simulink model "Copy_of_InvertedPendulumSimLuenberger"  (Simulink 9.2)
settings: Solver=ode5  StartTime=0.0  StopTime=30  FixedStep=0.01  RelTol=1e-3  AbsTol=1e-6
PreLoadFcn:
  | InvertedPendulumSimLuenbergerInit
InitFcn:
  | clear PlotPendulum
values from neighbouring files (symbols this model uses):
  A = [0, 1,          0,              0 ... (first row only)    [InvertedPendulumSimLuenbergerInit.m]    (also in aufgabe81.m = [0, -1; 1, -2]; aufgabe82.m = [0, 1; -1, 1])
  B = [ 0; J/d; 0; -mp*l/d]    [InvertedPendulumSimLuenbergerInit.m]    (also in aufgabe81.m = [0; 0.5]; aufgabe82.m = [0; 0.5])
  C = [ 1 0 0 0 ... (first row only)    [InvertedPendulumSimLuenbergerInit.m]    (also in aufgabe81.m = [0, 1]; aufgabe82.m = [1, 0])
  eta = 1.05    [InvertedPendulumSimLuenbergerInit.m]
  K = place(A,B,poles)    [InvertedPendulumSimLuenbergerInit.m]    (also in aufgabe82.m = place(A, B, [-3, -4]))
  kcw = 3    [InvertedPendulumSimLuenbergerInit.m]
  kem = 7    [InvertedPendulumSimLuenbergerInit.m]
  ksu = 1.3    [InvertedPendulumSimLuenbergerInit.m]
  kvw = 3    [InvertedPendulumSimLuenbergerInit.m]
  L = place(A', C', 2 * poles)'    [InvertedPendulumSimLuenbergerInit.m]    (also in aufgabe81.m = Lt'; aufgabe82.m = Lt')
  sigmaCart = 0    [InvertedPendulumSimLuenbergerInit.m]
  sigmaPend = 0    [InvertedPendulumSimLuenbergerInit.m]
  Td = 0    [InvertedPendulumSimLuenbergerInit.m]
  vmax = 5    [InvertedPendulumSimLuenbergerInit.m]
  x0 = [0; 0; pi-0.01; 0]    [InvertedPendulumSimLuenbergerInit.m]    (also in aufgabe81.m = [ -1; 1]; aufgabe82.m = [ -1; 1])
  x0hat = [0; 0; pi; 0]    [InvertedPendulumSimLuenbergerInit.m]    (also in aufgabe81.m = [ -2; 2]; aufgabe82.m = [ -2; 2])
  xmax = 0.4    [InvertedPendulumSimLuenbergerInit.m]
undefined symbols (not defined in the file or in its folder): fc, fp, Fs, g, J, l, M, m, mp, PlotPendulum, sgn, Ts
undefined symbols (not defined in the file): angleSZ
libraries: simulink x2
settings Model: LogicAnalyzerSignalOrdering=3f8627a9-a3d2-4771-9af9-cb62c719a4c2,aa08fdaf-5472-4d0b-8e2c-dcdd649b45f6,f94730cb-f55a-4896-8059-4683a2930ab6,1e4896a6-91b5-40dd-8c6c-ecf390694b00  Creator=jims  LastModifiedBy=root  ExtModeTrigDuration=12000  ExtModeTrigLevel=0.400000
settings SolverCC: AutoScaleAbsTol=off
settings DataIOCC: ExternalInput=[]  InitialState=[]  LimitDataPoints=off  MaxDataPoints=5000  SignalLoggingSaveFormat=Dataset  SaveOutput=off  SaveTime=off  SignalLoggingName=sigsOut
settings OptimizationCC: BooleanDataType=off  InitFltsAndDblsToZero=on
settings DebuggingCC: SaveWithParameterizedLinksMsg=none  SignalResolutionControl=TryResolveAllWithWarning  MultiTaskDSMMsg=warning  MultiTaskCondExecSysMsg=none  IntegerOverflowMsg=none  StateNameClashWarn=none  IntegerSaturationMsg=none
settings HardwareCC: TargetBitPerLong=64  TargetBitPerPointer=64  TargetBitPerSizeT=64  TargetBitPerPtrDiffT=64  TargetLongLongMode=on  TargetIntDivRoundTo=Zero  TargetEndianess=LittleEndian  TargetWordSize=64  TargetHWDeviceType=MATLAB Host  ProdEqTarget=off
settings SFSimCC: SimUseLocalCustomCode=on  SimParseCustomCode=off
settings RTWCC: SystemTargetFile=rtwin.tlc  TemplateMakefile=rtwin.tmf  RTWUseLocalCustomCode=on
settings TargetCC: TargetFcnLib=ansi_tfl_tmw.mat  ModelReferenceCompliant=off  CompOptLevelCompliant=off  GeneratePreprocessorConditionals=Use local settings  PreserveStateflowLocalDataDimensions=off
settings CustomProperty: DataType=string  Value=on
settings ConfigComp: CovExternalEMLEnable=on

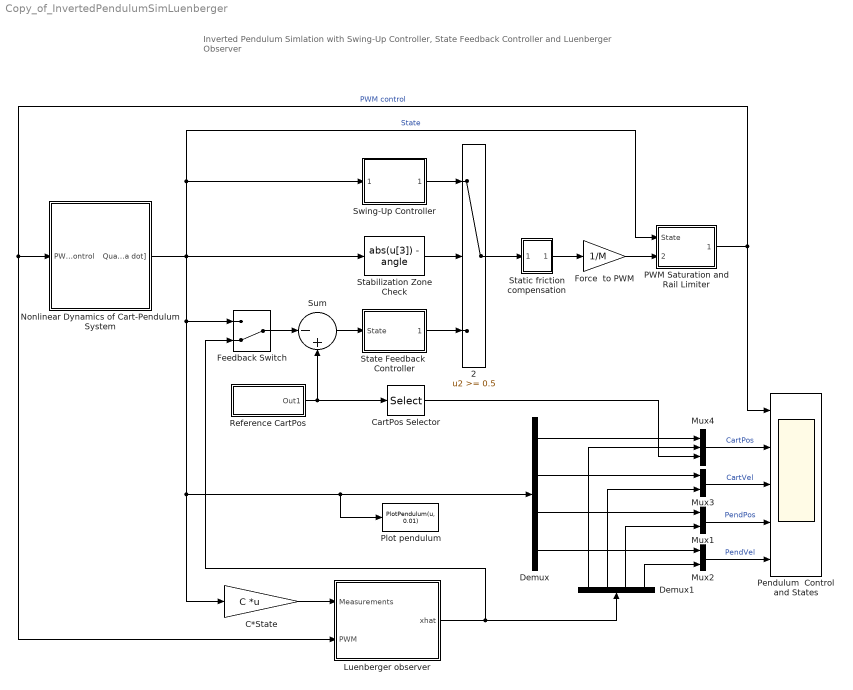
== system Copy_of_InvertedPendulumSimLuenberger ==
  note: Inverted Pendulum Simlation with
      | Swing-Up Controller, State Feedback Controller and
      | Luenberger Observer
  2 : Switch  Threshold=0.5  SaturateOnIntegerOverflow=on  InputSameDT=on
  C*State : Gain  Gain=C  Multiplication=Matrix(K*u) (u vector)
  CartPos Selector : Selector  InputPortWidth=4  IndexOptions=Index vector (dialog)  Indices=[1]  OutputSizes=1
  Demux : Demux
  Demux1 : Demux
  Feedback Switch : ManualSwitch  CurrentSetting=0
  Force  to PWM : Gain  Gain=1/M  SaturateOnIntegerOverflow=on  OutDataTypeStr=Inherit: Same as input  ParamDataTypeStr=Inherit: Same as input
  Luenberger observer : Subsystem
  Mux1 : Mux  Inputs=2
  Mux2 : Mux  Inputs=2
  Mux3 : Mux  Inputs=2
  Mux4 : Mux  Inputs=3
  Nonlinear Dynamics of Cart-Pendulum System : Subsystem  mask(Simulation of Pendulum Dynamics){}
      mask Display: plot(0,0,100,100,[40,48,48,40,40],[60,60,49,49,60],[37,44],[9,54],[100,8,4,1,0,100,100,0,40,100,100,0,0,40],[44,44,44,44,45,46,45,44,45,45,43,43,46,46],[100,48],[55,55],[0,40],[55,55])
  PWM Saturation and Rail Limiter : Subsystem  mask(State feedback controller){}
      mask Display: plot(0,0,100,100,[10,90,90,10],[52,52,50,50],[30,30],[52,60],[70,68,68,70,70],[60,60,52,52,60],[30,32,32,30],[52,52,60,60])
  Pendulum  Control and States : Scope  NumInputPorts=5
  Plot pendulum : MATLABFcn  MATLABFcn=PlotPendulum(u, 0.01)  OutputDimensions=0
  Reference CartPos : Subsystem  mask{Sine=off, Square=on, Sawtooth=off, Amplitude=0, Frequency=0.05}
      mask Display: disp('Generator')
  Stabilization Zone Check : Fcn  Expr=abs(u[3]) - angle  mask(Stabilization zone check){angle=angleSZ}
      mask prompts: angle "stabilization zone angle [rad]"
      mask help: Check if pendulum is insidde stabilization zone: abs(theta) <= angle
      mask Display: plot(0,0,100,100,[40,60,80,83,80,60,40,20,17,20,40],[89,89,80,70,60,51,51,60,69,80,90],[83,50,17],[70,8,68])
  State Feedback  Controller : Subsystem  mask(State feedback controller){}
      mask Display: plot(0,0,100,100,[40,30,20],[87,85,80],[46,54,54,46,46],[90,90,80,80,90],[46,45,45,46,54,55,55,54,46],[78,80,90,91,91,90,80,78,78],[51,51,49,49],[78,10,10,78],[90,80,70,60],[70,80,85,88],[20,10],[80,70],[20,20,15],[73,80,80],[85,80,80],[80,80,74])
  Static friction compensation : Subsystem  AncestorBlock=simulink/Discontinuities/Coulomb & Viscous Friction  mask(Static Friction){f=Fs}
      mask prompts: f "Static friction (f)"
      mask help:
      | A discontinuity offset at zero models static friction
      | y = u + sgn(u)*f
      mask Display: plot([-1 0 0 1],[-f-1, -f, f, 1+f],[-1 1],[0 0],[0 0],[-f,f])
  Sum : Sum  Inputs=|-+  SaturateOnIntegerOverflow=on
  Swing-Up Controller : Subsystem  mask(Swing-up Controller){}
      mask Display: plot(0,0,100,100,[20,20],[12,87],[93,90,90,93,7],[50,46,54,50,50],[20,22,18,20],[87,80,80,88],[80,80,75,75,71,71,65,65,60,60,49,49,40,40,20],[50,40,40,60,60,50,50,80,80,20,21,80,80,21,20])
  wires:
  Mux4/1 -> Pendulum  Control and States/2  "CartPos"
  Mux3/1 -> Pendulum  Control and States/3  "CartVel"
  Mux1/1 -> Pendulum  Control and States/4  "PendPos"
  Mux2/1 -> Pendulum  Control and States/5  "PendVel"
  Demux/4 -> Mux2/1
  Demux/3 -> Mux1/1
  Demux/2 -> Mux3/1
  Demux/1 -> Mux4/1
  Demux1/1 -> Mux4/2
  Demux1/2 -> Mux3/2
  Demux1/3 -> Mux1/2
  Demux1/4 -> Mux2/2
  Luenberger observer/1(xhat) -> Demux1/1, Feedback Switch/2
  Nonlinear Dynamics of Cart-Pendulum System/1(Quantizied state [x; x dot; theta; theta dot]) -> Swing-Up Controller/1(States), PWM Saturation and Rail Limiter/1(State), Demux/1, Plot pendulum/1, C*State/1, Feedback Switch/1, Stabilization Zone Check/1  "State"
  Reference CartPos/1(Out1) -> CartPos Selector/1, Sum/2
  Stabilization Zone Check/1 -> 2/2
  2/1 -> Static friction compensation/1(In1)
  Swing-Up Controller/1(Control) -> 2/1
  Static friction compensation/1(Out1) -> Force  to PWM/1
  Sum/1 -> State Feedback  Controller/1(State)
  CartPos Selector/1 -> Mux4/3
  State Feedback  Controller/1(Control input) -> 2/3
  Force  to PWM/1 -> PWM Saturation and Rail Limiter/2(Control input in)
  PWM Saturation and Rail Limiter/1(Control input out) -> Pendulum  Control and States/1, Luenberger observer/2(PWM), Nonlinear Dynamics of Cart-Pendulum System/1(PWM control)  "PWM control"
  Feedback Switch/1 -> Sum/1
  C*State/1 -> Luenberger observer/1(Measurements)

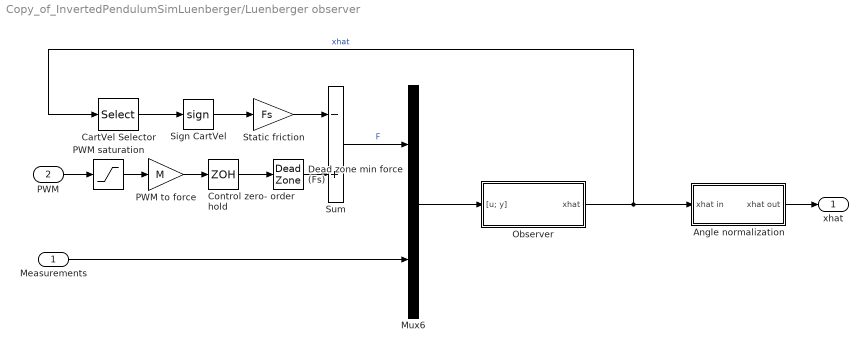
== system Copy_of_InvertedPendulumSimLuenberger/Luenberger observer ==
  Measurements : Inport
  PWM : Inport  Port=2
  Angle normalization : Subsystem
  CartVel Selector : Selector  InputPortWidth=4  IndexOptions=Index vector (dialog)  Indices=[2]  OutputSizes=1
  Control zero- order hold : ZeroOrderHold  SampleTime=Ts
  Dead zone min force (Fs) : DeadZone  LowerValue=-Fs  UpperValue=Fs  SaturateOnIntegerOverflow=on
  Mux6 : Mux  Inputs=2
  Observer : Subsystem
  PWM saturation : Saturate
  PWM to force : Gain  Gain=M  SaturateOnIntegerOverflow=on  OutDataTypeStr=Inherit: Same as input  ParamDataTypeStr=Inherit: Same as input
  Sign CartVel : Signum
  Static friction : Gain  Gain=Fs  SaturateOnIntegerOverflow=on  OutDataTypeStr=Inherit: Same as input  ParamDataTypeStr=Inherit: Same as input
  Sum : Sum  Inputs=-+  SaturateOnIntegerOverflow=on  InputSameDT=on  OutDataTypeStr=Inherit: Same as first input
  xhat : Outport
  wires:
  Measurements/1 -> Mux6/2
  Angle normalization/1(xhat out) -> xhat/1
  Mux6/1 -> Observer/1("[u; y]")
  Observer/1(xhat) -> CartVel Selector/1, Angle normalization/1(xhat in)  "xhat"
  CartVel Selector/1 -> Sign CartVel/1
  Static friction/1 -> Sum/1
  PWM to force/1 -> Control zero- order hold/1
  Control zero- order hold/1 -> Dead zone min force (Fs)/1
  Dead zone min force (Fs)/1 -> Sum/2
  Sign CartVel/1 -> Static friction/1
  PWM saturation/1 -> PWM to force/1
  Sum/1 -> Mux6/1  "F"
  PWM/1 -> PWM saturation/1

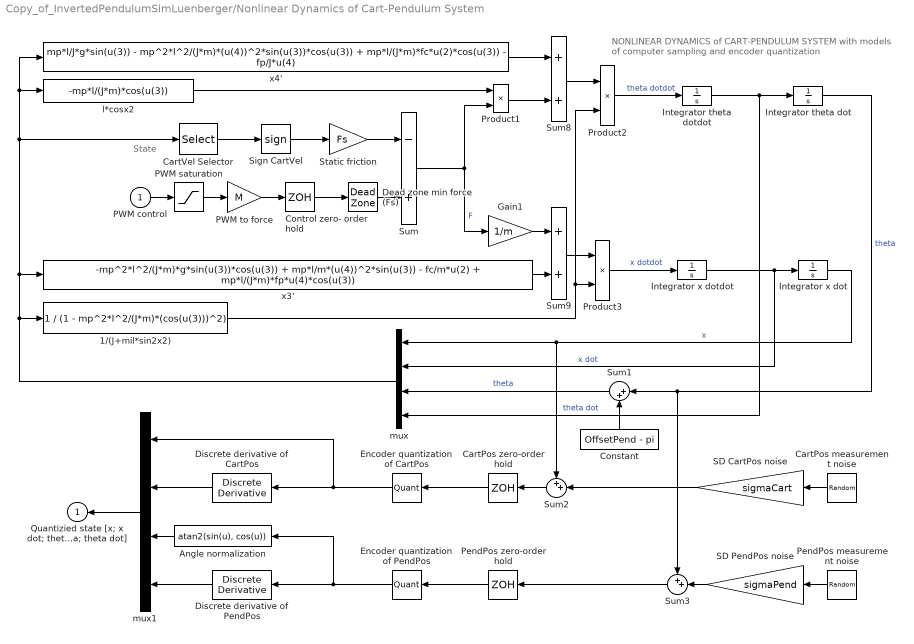
== system Copy_of_InvertedPendulumSimLuenberger/Nonlinear Dynamics of Cart-Pendulum System ==
  note: NONLINEAR DYNAMICS of CART-PENDULUM
      | SYSTEM with models of computer sampling
      | and encoder quantization
  note: State
  PWM control : Inport
  1/(J+mil*sin2x2) : Fcn  Expr=1 / (1 - mp^2*l^2/(J*m)*(cos(u(3)))^2)
  Angle normalization : Fcn  Expr=atan2(sin(u), cos(u))
  CartPos measurement noise : RandomNumber  SampleTime=Ts
  CartPos zero-order hold : ZeroOrderHold  SampleTime=Ts
  CartVel Selector : Selector  InputPortWidth=4  IndexOptions=Index vector (dialog)  Indices=[2]  OutputSizes=1
  Constant : Constant  Value=OffsetPend - pi
  Control zero- order hold : ZeroOrderHold  SampleTime=Ts
  Dead zone min force (Fs) : DeadZone  LowerValue=-Fs  UpperValue=Fs  SaturateOnIntegerOverflow=on
  Discrete derivative of CartPos : simulink/Discrete/Discrete Derivative  gainval=1.0  ICPrevScaledInput=x0(1)/Ts  OutMin=[]  OutMax=[]  OutDataType=sfix(16)  OutScaling=2^-10  DoSatur=off
  Discrete derivative of PendPos : simulink/Discrete/Discrete Derivative  gainval=1.0  ICPrevScaledInput=x0(3)/Ts  OutMin=[]  OutMax=[]  OutDataType=sfix(16)  OutScaling=2^-10  DoSatur=off
  Encoder quantization of CartPos : Quantizer  QuantizationInterval=ResCartEnc
  Encoder quantization of PendPos : Quantizer  QuantizationInterval=ResPendEnc
  Gain1 : Gain  Gain=1/m  SaturateOnIntegerOverflow=on  OutDataTypeStr=Inherit: Same as input  ParamDataTypeStr=Inherit: Same as input
  Integrator theta dot : Integrator  InitialCondition=x0(3)
  Integrator theta dotdot : Integrator  InitialCondition=x0(4)
  Integrator x dot : Integrator  InitialCondition=x0(1)
  Integrator x dotdot : Integrator  InitialCondition=x0(2)
  PWM saturation : Saturate
  PWM to force : Gain  Gain=M  SaturateOnIntegerOverflow=on  OutDataTypeStr=Inherit: Same as input  ParamDataTypeStr=Inherit: Same as input
  PendPos measurement noise : RandomNumber  SampleTime=Ts
  PendPos zero-order hold : ZeroOrderHold  SampleTime=Ts
  Product1 : Product  SaturateOnIntegerOverflow=on  InputSameDT=on  OutDataTypeStr=Inherit: Same as first input
  Product2 : Product  SaturateOnIntegerOverflow=on  InputSameDT=on  OutDataTypeStr=Inherit: Same as first input
  Product3 : Product  SaturateOnIntegerOverflow=on  InputSameDT=on  OutDataTypeStr=Inherit: Same as first input
  SD CartPos noise : Gain  Gain=sigmaCart  SaturateOnIntegerOverflow=on  OutDataTypeStr=Inherit: Same as input  ParamDataTypeStr=Inherit: Same as input
  SD PendPos noise : Gain  Gain=sigmaPend  SaturateOnIntegerOverflow=on  OutDataTypeStr=Inherit: Same as input  ParamDataTypeStr=Inherit: Same as input
  Sign CartVel : Signum
  Static friction : Gain  Gain=Fs  SaturateOnIntegerOverflow=on  OutDataTypeStr=Inherit: Same as input  ParamDataTypeStr=Inherit: Same as input
  Sum : Sum  Inputs=-+  SaturateOnIntegerOverflow=on  InputSameDT=on  OutDataTypeStr=Inherit: Same as first input
  Sum1 : Sum  Inputs=|++  SaturateOnIntegerOverflow=on  InputSameDT=on  OutDataTypeStr=Inherit: Same as first input
  Sum2 : Sum  Inputs=++|  SaturateOnIntegerOverflow=on  InputSameDT=on  OutDataTypeStr=Inherit: Same as first input
  Sum3 : Sum  Inputs=++|  SaturateOnIntegerOverflow=on  InputSameDT=on  OutDataTypeStr=Inherit: Same as first input
  Sum8 : Sum  SaturateOnIntegerOverflow=on  InputSameDT=on  OutDataTypeStr=Inherit: Same as first input
  Sum9 : Sum  SaturateOnIntegerOverflow=on  InputSameDT=on  OutDataTypeStr=Inherit: Same as first input
  l*cosx2 : Fcn  Expr=-mp*l/(J*m)*cos(u(3))
  mux : Mux
  mux1 : Mux
  x3' : Fcn  Expr=-mp^2*l^2/(J*m)*g*sin(u(3))*cos(u(3)) + mp*l/m*(u(4))^2*sin(u(3)) - fc/m*u(2) + mp*l/(J*m)*fp*u(4)*cos(u(3))
  x4' : Fcn  Expr=mp*l/J*g*sin(u(3)) - mp^2*l^2/(J*m)*(u(4))^2*sin(u(3))*cos(u(3)) + mp*l/(J*m)*fc*u(2)*cos(u(3)) - fp/J*u(4)
  Quantizied state [x; x dot; theta; theta dot] : Outport  InitialOutput=0
  wires:
  CartPos zero-order hold/1 -> Encoder quantization of CartPos/1
  mux/1 -> 1/(J+mil*sin2x2)/1, x3'/1, l*cosx2/1, x4'/1, CartVel Selector/1
  Encoder quantization of CartPos/1 -> mux1/1, Discrete derivative of CartPos/1
  Integrator theta dotdot/1 -> mux/4, Integrator theta dot/1  "theta dot"
  l*cosx2/1 -> Product1/1
  Product1/1 -> Sum8/2
  Product2/1 -> Integrator theta dotdot/1  "theta dotdot"
  Product3/1 -> Integrator x dotdot/1  "x dotdot"
  Sum9/1 -> Product3/1
  Integrator x dotdot/1 -> Integrator x dot/1, mux/2  "x dot"
  Sum/1 -> Product1/2, Gain1/1  "F"
  x3'/1 -> Sum9/2
  Gain1/1 -> Sum9/1
  Sum8/1 -> Product2/1
  x4'/1 -> Sum8/1
  CartVel Selector/1 -> Sign CartVel/1
  Static friction/1 -> Sum/1
  1/(J+mil*sin2x2)/1 -> Product2/2, Product3/2
  PWM control/1 -> PWM saturation/1
  PWM to force/1 -> Control zero- order hold/1
  Control zero- order hold/1 -> Dead zone min force (Fs)/1
  PendPos zero-order hold/1 -> Encoder quantization of PendPos/1
  Encoder quantization of PendPos/1 -> Angle normalization/1, Discrete derivative of PendPos/1
  Discrete derivative of PendPos/1 -> mux1/4
  Angle normalization/1 -> mux1/3
  Discrete derivative of CartPos/1 -> mux1/2
  mux1/1 -> Quantizied state [x; x dot; theta; theta dot]/1
  Sum2/1 -> CartPos zero-order hold/1
  SD CartPos noise/1 -> Sum2/2
  CartPos measurement noise/1 -> SD CartPos noise/1
  Sum3/1 -> PendPos zero-order hold/1
  SD PendPos noise/1 -> Sum3/2
  PendPos measurement noise/1 -> SD PendPos noise/1
  Dead zone min force (Fs)/1 -> Sum/2
  Sign CartVel/1 -> Static friction/1
  Integrator theta dot/1 -> Sum3/1, Sum1/1  "theta"
  Integrator x dot/1 -> mux/1, Sum2/1  "x"
  PWM saturation/1 -> PWM to force/1
  Sum1/1 -> mux/3  "theta"
  Constant/1 -> Sum1/2

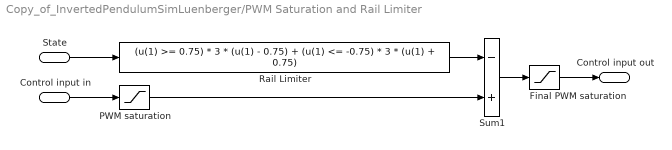
== system Copy_of_InvertedPendulumSimLuenberger/PWM Saturation and Rail Limiter ==
  State : Inport
  Control input in : Inport  Port=2
  Final PWM saturation : Saturate
  PWM saturation : Saturate
  Rail Limiter : Fcn  Expr=(u(1) >= 0.75) * 3 * (u(1) - 0.75) + (u(1) <= -0.75) * 3 * (u(1) + 0.75)
  Sum1 : Sum  Inputs=-+  SaturateOnIntegerOverflow=on  InputSameDT=on  OutDataTypeStr=Inherit: Same as first input
  Control input out : Outport  InitialOutput=0
  wires:
  State/1 -> Rail Limiter/1
  Rail Limiter/1 -> Sum1/1
  Control input in/1 -> PWM saturation/1
  Sum1/1 -> Final PWM saturation/1
  PWM saturation/1 -> Sum1/2
  Final PWM saturation/1 -> Control input out/1

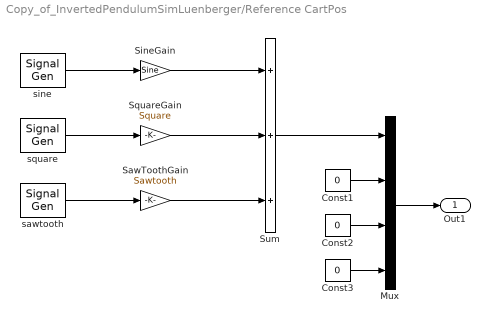
== system Copy_of_InvertedPendulumSimLuenberger/Reference CartPos ==
  Const1 : Constant  Value=0
  Const2 : Constant  Value=0
  Const3 : Constant  Value=0
  Mux : Mux
  SawToothGain : Gain  Gain=Sawtooth  SaturateOnIntegerOverflow=on  OutDataTypeStr=Inherit: Same as input  ParamDataTypeStr=Inherit: Same as input
  SineGain : Gain  Gain=Sine  SaturateOnIntegerOverflow=on  OutDataTypeStr=Inherit: Same as input  ParamDataTypeStr=Inherit: Same as input
  SquareGain : Gain  Gain=Square  SaturateOnIntegerOverflow=on  OutDataTypeStr=Inherit: Same as input  ParamDataTypeStr=Inherit: Same as input
  Sum : Sum  Inputs=+++  SaturateOnIntegerOverflow=on  InputSameDT=on  OutDataTypeStr=Inherit: Same as first input
  sawtooth : SignalGenerator  WaveForm=sawtooth  Amplitude=Amplitude  Frequency=Frequency
  sine : SignalGenerator  Amplitude=Amplitude  Frequency=Frequency
  square : SignalGenerator  WaveForm=square  Amplitude=Amplitude  Frequency=Frequency
  Out1 : Outport  InitialOutput=0
  wires:
  SawToothGain/1 -> Sum/3
  SquareGain/1 -> Sum/2
  SineGain/1 -> Sum/1
  sawtooth/1 -> SawToothGain/1
  square/1 -> SquareGain/1
  sine/1 -> SineGain/1
  Const2/1 -> Mux/3
  Const3/1 -> Mux/4
  Mux/1 -> Out1/1
  Const1/1 -> Mux/2
  Sum/1 -> Mux/1

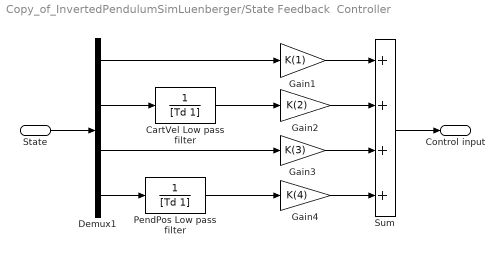
== system Copy_of_InvertedPendulumSimLuenberger/State Feedback  Controller ==
  State : Inport
  CartVel Low pass filter : TransferFcn  Denominator=[Td 1]
  Demux1 : Demux
  Gain1 : Gain  Gain=K(1)  SaturateOnIntegerOverflow=on  OutDataTypeStr=Inherit: Same as input  ParamDataTypeStr=Inherit: Same as input
  Gain2 : Gain  Gain=K(2)  SaturateOnIntegerOverflow=on  OutDataTypeStr=Inherit: Same as input  ParamDataTypeStr=Inherit: Same as input
  Gain3 : Gain  Gain=K(3)  SaturateOnIntegerOverflow=on  OutDataTypeStr=Inherit: Same as input  ParamDataTypeStr=Inherit: Same as input
  Gain4 : Gain  Gain=K(4)  SaturateOnIntegerOverflow=on  OutDataTypeStr=Inherit: Same as input  ParamDataTypeStr=Inherit: Same as input
  PendPos Low pass filter : TransferFcn  Denominator=[Td 1]
  Sum : Sum  Inputs=++++  SaturateOnIntegerOverflow=on  InputSameDT=on  OutDataTypeStr=Inherit: Same as first input
  Control input : Outport  InitialOutput=0
  wires:
  Demux1/1 -> Gain1/1
  Gain1/1 -> Sum/1
  Gain2/1 -> Sum/2
  Demux1/2 -> CartVel Low pass filter/1
  Gain3/1 -> Sum/3
  Demux1/3 -> Gain3/1
  Gain4/1 -> Sum/4
  Demux1/4 -> PendPos Low pass filter/1
  Sum/1 -> Control input/1
  State/1 -> Demux1/1
  PendPos Low pass filter/1 -> Gain4/1
  CartVel Low pass filter/1 -> Gain2/1

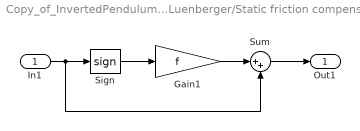
== system Copy_of_InvertedPendulumSimLuenberger/Static friction compensation ==
  In1 : Inport
  Gain1 : Gain  Gain=f  SaturateOnIntegerOverflow=on  OutDataTypeStr=Inherit: Same as input  ParamDataTypeStr=Inherit: Same as input
  Sign : Signum
  Sum : Sum  Inputs=|++  SaturateOnIntegerOverflow=on  InputSameDT=on  OutDataTypeStr=Inherit: Same as first input
  Out1 : Outport
  wires:
  Sign/1 -> Gain1/1
  In1/1 -> Sign/1, Sum/2
  Gain1/1 -> Sum/1
  Sum/1 -> Out1/1

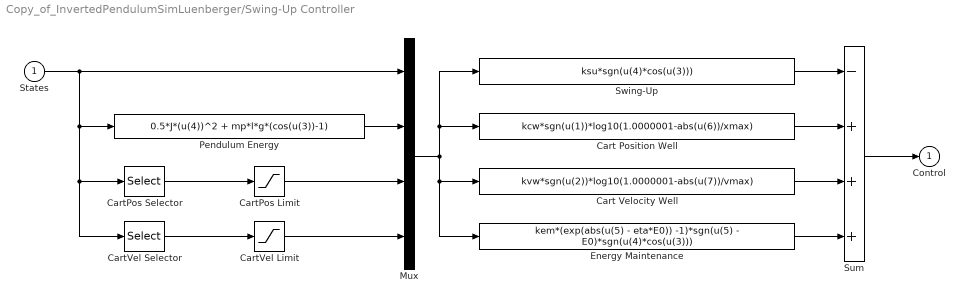
== system Copy_of_InvertedPendulumSimLuenberger/Swing-Up Controller ==
  States : Inport
  Cart Position Well : Fcn  Expr=kcw*sgn(u(1))*log10(1.0000001-abs(u(6))/xmax)
  Cart Velocity Well : Fcn  Expr=kvw*sgn(u(2))*log10(1.0000001-abs(u(7))/vmax)
  CartPos Limit : Saturate  UpperLimit=xmax  LowerLimit=-xmax
  CartPos Selector : Selector  InputPortWidth=4  IndexOptions=Index vector (dialog)  Indices=[1]  OutputSizes=1
  CartVel Limit : Saturate  UpperLimit=vmax  LowerLimit=-vmax
  CartVel Selector : Selector  InputPortWidth=4  IndexOptions=Index vector (dialog)  Indices=[2]  OutputSizes=1
  Energy Maintenance : Fcn  Expr=kem*(exp(abs(u(5) - eta*E0)) -1)*sgn(u(5) - E0)*sgn(u(4)*cos(u(3)))
  Mux : Mux
  Pendulum Energy : Fcn  Expr=0.5*J*(u(4))^2 + mp*l*g*(cos(u(3))-1)
  Sum : Sum  Inputs=-+++  SaturateOnIntegerOverflow=on
  Swing-Up : Fcn  Expr=ksu*sgn(u(4)*cos(u(3)))
  Control : Outport  InitialOutput=0
  wires:
  States/1 -> Mux/1, Pendulum Energy/1, CartPos Selector/1, CartVel Selector/1
  Pendulum Energy/1 -> Mux/2
  CartPos Selector/1 -> CartPos Limit/1
  CartPos Limit/1 -> Mux/3
  CartVel Selector/1 -> CartVel Limit/1
  CartVel Limit/1 -> Mux/4
  Mux/1 -> Swing-Up/1, Cart Position Well/1, Cart Velocity Well/1, Energy Maintenance/1
  Sum/1 -> Control/1
  Swing-Up/1 -> Sum/1
  Cart Position Well/1 -> Sum/2
  Cart Velocity Well/1 -> Sum/3
  Energy Maintenance/1 -> Sum/4

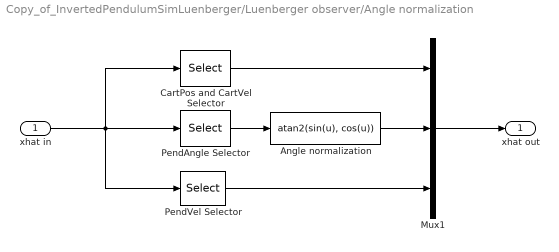
== system Copy_of_InvertedPendulumSimLuenberger/Luenberger observer/Angle normalization ==
  xhat in : Inport
  Angle normalization : Fcn  Expr=atan2(sin(u), cos(u))
  CartPos and CartVel Selector : Selector  InputPortWidth=4  IndexOptions=Index vector (dialog)  Indices=[1 2]  OutputSizes=1
  Mux1 : Mux  Inputs=3
  PendAngle Selector : Selector  InputPortWidth=4  IndexOptions=Index vector (dialog)  Indices=[3]  OutputSizes=1
  PendVel Selector : Selector  InputPortWidth=4  IndexOptions=Index vector (dialog)  Indices=[4]  OutputSizes=1
  xhat out : Outport
  wires:
  xhat in/1 -> PendAngle Selector/1, PendVel Selector/1, CartPos and CartVel Selector/1
  PendAngle Selector/1 -> Angle normalization/1
  CartPos and CartVel Selector/1 -> Mux1/1
  Angle normalization/1 -> Mux1/2
  PendVel Selector/1 -> Mux1/3
  Mux1/1 -> xhat out/1

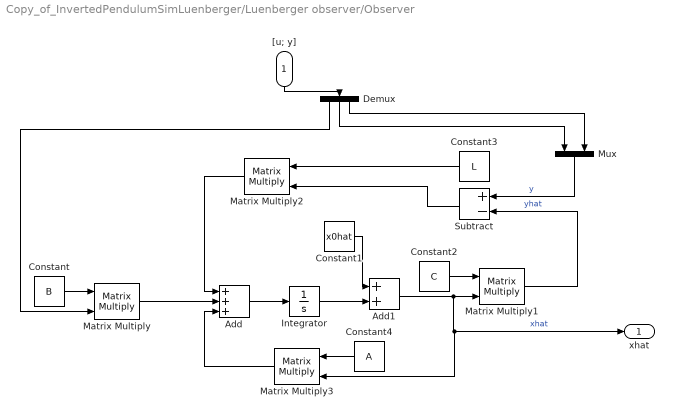
== system Copy_of_InvertedPendulumSimLuenberger/Luenberger observer/Observer ==
  "[u; y]" : Inport
  Add : Sum  Inputs=+++
  Add1 : Sum
  Constant : Constant  Value=B  VectorParams1D=off
  Constant1 : Constant  Value=x0hat
  Constant2 : Constant  Value=C
  Constant3 : Constant  Value=L
  Constant4 : Constant  Value=A
  Demux : Demux  Outputs=3
  Integrator : Integrator
  Matrix Multiply{,1..3} (4 alike) : Product  Multiplication=Matrix(*)
  Mux : Mux  Inputs=2
  Subtract : Sum  Inputs=+-
  xhat : Outport
  wires:
  "[u; y]"/1 -> Demux/1
  Demux/2 -> Mux/1
  Mux/1 -> Subtract/1  "y"
  Constant/1 -> Matrix Multiply/1
  Matrix Multiply/1 -> Add/2
  Add/1 -> Integrator/1
  Integrator/1 -> Add1/2
  Constant1/1 -> Add1/1
  Add1/1 -> Matrix Multiply3/2, xhat/1, Matrix Multiply1/2  "xhat"
  Constant2/1 -> Matrix Multiply1/1
  Matrix Multiply1/1 -> Subtract/2  "yhat"
  Constant3/1 -> Matrix Multiply2/1
  Subtract/1 -> Matrix Multiply2/2
  Matrix Multiply2/1 -> Add/1
  Constant4/1 -> Matrix Multiply3/1
  Matrix Multiply3/1 -> Add/3
  Demux/1 -> Matrix Multiply/2
  Demux/3 -> Mux/2
